simulink model "Thermal_first"  (R2021b)
settings: Solver=ode23t  StartTime=0.0  StopTime=1305  MaxStep=1e-3  RelTol=1e-3
libraries: simulink x2
settings Model: Creator=alexey  LastModifiedBy=alexey
settings SolverCC: ZeroCrossControl=DisableAll

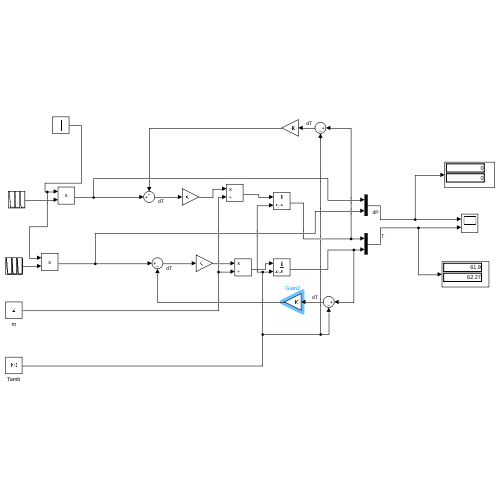
[thumbnail: Simulink's stored preview of the top-level diagram]
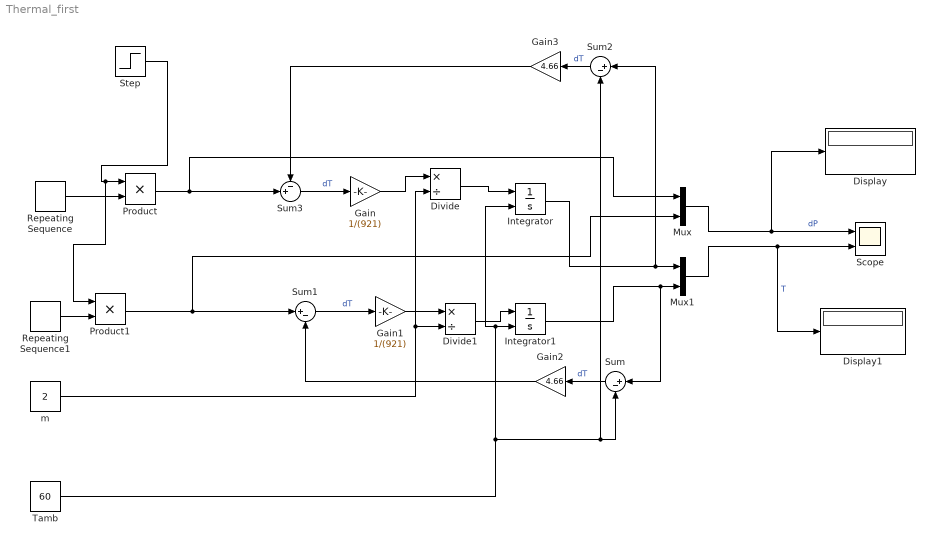
== system Thermal_first ==
  Display : Display
  Display1 : Display
  Divide : Product  Inputs=*/
  Divide1 : Product  Inputs=*/
  Gain : Gain  Gain=1/(921)
  Gain1 : Gain  Gain=1/(921)
  Gain2 : Gain  Gain=4.66
  Gain3 : Gain  Gain=4.66
  Integrator : Integrator  InitialConditionSource=external
  Integrator1 : Integrator  InitialConditionSource=external
  Mux : Mux  Inputs=2
  Mux1 : Mux  Inputs=2
  Product : Product
  Product1 : Product
  Repeating Sequence : simulink/Sources/Repeating Sequence  rep_seq_t=[0 5 10 15 20 25 30 35 40 40.1 140.1]  rep_seq_y=[849 849 849 849 592 332 128 62 62 0 0]
  Repeating Sequence1 : simulink/Sources/Repeating Sequence  rep_seq_t=[0 5 10 15 20 25 30 35 40 40.1 140.1]  rep_seq_y=[1480 1187 1028 849 592 332 128 62 62 0 0]
  Scope : Scope  NumInputPorts=2
  Step : Step  Time=400  Before=1  After=0  SampleTime=0
  Sum : Sum  Inputs=|+-
  Sum1 : Sum  Inputs=|+-
  Sum2 : Sum  Inputs=|+-
  Sum3 : Sum  Inputs=-+|
  Tamb : Constant  Value=60  VectorParams1D=off
  m : Constant  Value=2
  wires:
  Product/1 -> Mux/1, Sum3/2
  Gain/1 -> Divide/1
  Integrator1/1 -> Sum/1, Mux1/2
  Gain1/1 -> Divide1/1
  Product1/1 -> Sum1/1, Mux/2
  Mux/1 -> Display/1, Scope/1  "dP"
  Mux1/1 -> Display1/1, Scope/2  "T"
  Sum/1 -> Gain2/1  "dT"
  Sum1/1 -> Gain1/1  "dT"
  Gain2/1 -> Sum1/2
  Sum2/1 -> Gain3/1  "dT"
  Tamb/1 -> Sum2/2, Sum/2, Integrator1/2, Integrator/2
  Integrator/1 -> Sum2/1, Mux1/1
  Sum3/1 -> Gain/1  "dT"
  Gain3/1 -> Sum3/1
  Step/1 -> Product1/1, Product/1
  Repeating Sequence/1 -> Product/2
  Repeating Sequence1/1 -> Product1/2
  Divide/1 -> Integrator/1
  Divide1/1 -> Integrator1/1
  m/1 -> Divide1/2, Divide/2
